simulink model "closed_loop"  (R2021b)
settings: Solver=ode4  StartTime=0.0  StopTime=5  FixedStep=0.01  RelTol=1e-3
values from neighbouring files (symbols this model uses):
  A = [0        0                     1               0 ... (first row only)    [IP.m]    (also in IP_experiment.m; IP_sim.m)
  B = [         0 ... (first row only)    [IP.m]    (also in IP_experiment.m; IP_sim.m)
  C = eye(4)    [IP.m]    (also in IP_experiment.m = [1 0 0 0; IP_sim.m = [1 0 0 0)
  D = zeros(4, 1)    [IP.m]    (also in IP_experiment.m = [0;0]; IP_sim.m = [0;0])
  x0 = [pos_init  angle_init  0   0]'    [IP.m]    (also in IP_experiment.m = [pos_init  angle_init      0.0     0.0]; IP_sim.m = [pos_init  angle_init      0.0     0.0])
  xd = [0.3          0.0      0   0]'    [IP.m]    (also in IP_experiment.m = [0.0    0.0]; IP_sim.m = [0.3    0.0])
undefined symbols (not defined in the file or in its folder): K
settings Model: Creator=yz  LastModifiedBy=yz

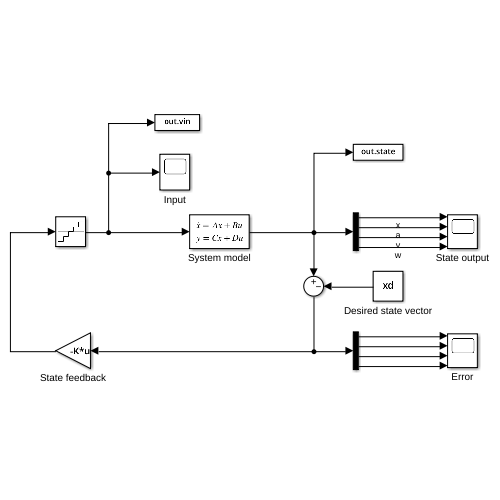
[thumbnail: Simulink's stored preview of the top-level diagram]
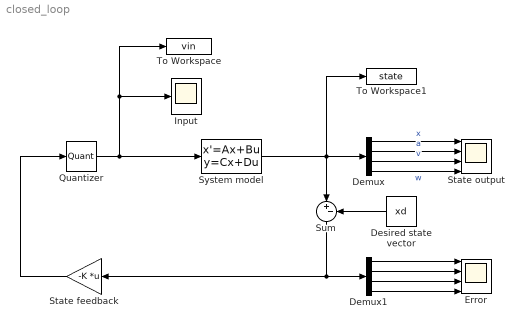
== system closed_loop ==
  Demux : Demux
  Demux1 : Demux
  Desired state vector : Constant  Value=xd  VectorParams1D=off
  Error : Scope  NumInputPorts=4
  Input : Scope
  Quantizer : Quantizer  QuantizationInterval=0.00031
  State feedback : Gain  Gain=-K  Multiplication=Matrix(K*u)
  State output : Scope  NumInputPorts=4
  Sum : Sum  Inputs=|+-
  System model : StateSpace  A=A  B=B  C=C  D=D  InitialCondition=x0
  To Workspace : ToWorkspace  VariableName=vin  SampleTime=-1
      settings: Save2DSignal=2-D array (concatenate along first dimension)
  To Workspace1 : ToWorkspace  VariableName=state  SampleTime=-1
  wires:
  Desired state vector/1 -> Sum/2
  Sum/1 -> State feedback/1, Demux1/1
  Demux/2 -> State output/2  "a"
  Demux/1 -> State output/1  "x"
  Demux/3 -> State output/3  "v"
  Demux/4 -> State output/4  "w"
  Demux1/1 -> Error/1
  Demux1/2 -> Error/2
  Demux1/3 -> Error/3
  Demux1/4 -> Error/4
  System model/1 -> Sum/1, To Workspace1/1, Demux/1
  State feedback/1 -> Quantizer/1
  Quantizer/1 -> Input/1, To Workspace/1, System model/1
